simulink model "LQR_sim_discrete"  (R2020b)
settings: Solver=FixedStepAuto  StartTime=0.0  StopTime=60  FixedStep=0.0001  RelTol=1e-3  EnableMultiTasking=on
values from neighbouring files (symbols this model uses):
  Theta1_0 = pi    (= 3.14159265359)    [simulation.m]
  Theta2_0 = -pi/2    (= -1.57079632679)    [simulation.m]
  Thetad1_0 = 0    [simulation.m]
  Thetad2_0 = 0    [simulation.m]
undefined symbols (not defined in the file or in its folder): Discrete, h, Kd, Q, R, Time
libraries: simulink x4, ctrlSharedLib x1
settings Model: Creator=rbabuska  LastModifiedBy=fabia
settings SolverCC: AutoInsertRateTranBlk=on
settings DataIOCC: LimitDataPoints=on  SaveFormat=Array  ReturnWorkspaceOutputs=off  SignalLoggingName=sigsOut
settings OptimizationCC: BooleanDataType=off  ExpressionDepthLimit=2147483647  InitFltsAndDblsToZero=on  LifeSpan=inf
settings DebuggingCC: SaveWithParameterizedLinksMsg=none  SignalResolutionControl=TryResolveAllWithWarning  MultiTaskDSMMsg=warning  MultiTaskCondExecSysMsg=none  AllowSymbolicDim=off  StateNameClashWarn=warning  SFUnexpectedBacktrackingDiag=warning  SFNoUnconditionalDefaultTransitionDiag=warning  SFExecutionAtInitializationDiag=none  ArithmeticOperatorsInVariantConditions=warning
settings HardwareCC: ProdBitPerPointer=32  ProdBitPerSizeT=32  ProdBitPerPtrDiffT=32  ProdLargestAtomicFloat=None  ProdIntDivRoundTo=Undefined  ProdEndianess=Unspecified  ProdWordSize=32  ProdHWDeviceType=32-bit Generic  TargetUnknown=on
settings ModelReferenceCC: PropagateSignalLabelsOutOfModel=off
settings SFSimCC: SimUseLocalCustomCode=off  CustomCodeUndefinedFunction=UseInterfaceOnly
settings RTWCC: RTWUseLocalCustomCode=off
settings CodeAppCC: StateflowObjectComments=on
settings GRTTargetCC: TargetFcnLib=ansi_tfl_tmw.mat  TargetLangStandard=C89/C90 (ANSI)  CombineOutputUpdateFcns=off  GRTInterface=on
settings ConfigComp: CovMetricSettings=dw  CovSaveCumulativeToWorkspaceVar=on  CovSaveSingleToWorkspaceVar=on  CovExternalEMLEnable=off

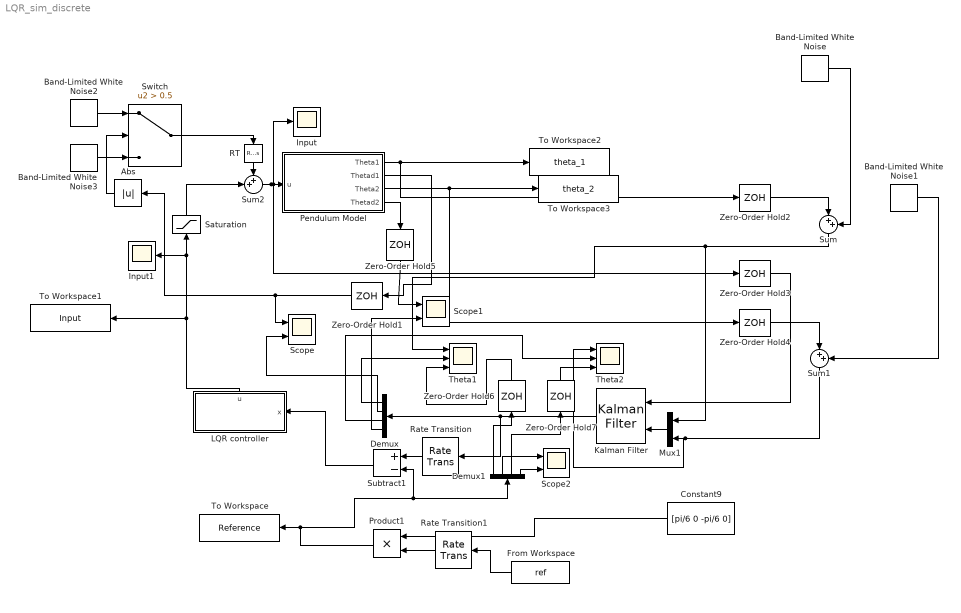
== system LQR_sim_discrete ==
  Abs : Abs
  Band-Limited White Noise : simulink/Sources/Band-Limited White Noise  Cov=R(1,1) * h  Ts=h  seed=[23341]
  Band-Limited White Noise1 : simulink/Sources/Band-Limited White Noise  Cov=R(2,2) * h  Ts=h  seed=[23546]
  Band-Limited White Noise2 : simulink/Sources/Band-Limited White Noise  Cov=Q*h  Ts=0.01  seed=[23341]
  Band-Limited White Noise3 : simulink/Sources/Band-Limited White Noise  Cov=Q*5  Ts=0.01  seed=[23341]
  Constant9 : Constant  Value=[pi/6 0 -pi/6 0]
  Demux : Demux
  Demux1 : Demux
  From Workspace : FromWorkspace  VariableName=ref  SampleTime=h
  Input : Scope
  Input1 : Scope
  Kalman Filter : ctrlSharedLib/Kalman Filter  TimeDomain=Discrete-Time  UseCurrentEstimator=on  ModelSource=LTI State-Space Variable  ModelSourceVariable=sysd  A=0.95  B=1  C=1  D=0  NumberOfStates=1  NumberOfInputs=1  NumberOfOutputs=1  InitialEstimateSource=Dialog  X0=0  P0=10  UseK=off  UseGH=off  NumberOfProcessNoiseInputs=1  G=1  TimeInvariantG=on  H=0  TimeInvariantH=on  Q=Q  TimeInvariantQ=on  R=R  TimeInvariantR=on  N=0  TimeInvariantN=on  AddInputPort=on  AddEnablePort=off  OutputEstimatedY=off  OutputP=off  Ts=-1
  LQR controller : Subsystem
      settings: PortSchema="{\"entries\":[{\"content\":{\"sides\":[{\"content\":{\"connectorIds\":[\"In1\"]},\"type\":\"ConnectorPlacement.EquallySpacedRectSide\",\"uuid\":\"a829bb76-8c32-4efb-bc1d-6bbdd337957d\"},{\"content\":{\"connectorIds\":[],\"side\":\"RIGHT\"},\"type\":\"ConnectorPlacement.EquallySpacedRectSide\",\"uuid\":\"eecab09d-eb4e-4271-bbad-67f1ecd3f7cb\"},{\"content\":{\"connectorIds\":[\"Out1\"],\"side\":\"TOP\"},\"type\":\"ConnectorPlacement.EquallySpacedRectSide\",\"uuid\":\"cb69e62e-93af-466c-bc77-09ee124a36c9\"},{\"content\":{\"connectorIds\":[],\"side\":\"HIDDEN\"},\"type\":\"ConnectorPlacement.EquallySpacedRectSide\",\"uuid\":\"8cf3d3f7-c3b5-449a-9c77-3afa19a1a637\"}]},\"type\":\"ConnectorPlacement.EquallySpacedConnector\",\"uuid\":\"e69d0e99-04d0-49a4-bcc0-927adbe84b1d\"}],\"packageUris\":[\"http://schema.mathworks.com/mf0/Connector/R2020b\"],\"version\":\"1.0\"}"
  Mux1 : Mux  Inputs=2
  Pendulum Model : Subsystem
  Product1 : Product
  RT : RateTransition  OutPortSampleTime=0.0001
  Rate Transition : RateTransition
  Rate Transition1 : RateTransition
  Saturation : Saturate  UpperLimit=1  LowerLimit=-1
  Scope : Scope  NumInputPorts=2
  Scope1 : Scope  NumInputPorts=2
  Scope2 : Scope  NumInputPorts=2
  Subtract1 : Sum  Inputs=+-
  Sum : Sum  Inputs=|++
  Sum1 : Sum  Inputs=|++
  Sum2 : Sum  Inputs=++|
  Switch : Switch  Criteria=u2 > Threshold  Threshold=0.5
  Theta1 : Scope  NumInputPorts=3
  Theta2 : Scope  NumInputPorts=3
  To Workspace : ToWorkspace  VariableName=Reference  SaveFormat=Timeseries  SampleTime=-1
  To Workspace1 : ToWorkspace  VariableName=Input  SaveFormat=Timeseries  SampleTime=-1
  To Workspace2 : ToWorkspace  VariableName=theta_1  SaveFormat=Timeseries  SampleTime=-1
  To Workspace3 : ToWorkspace  VariableName=theta_2  SaveFormat=Timeseries  SampleTime=-1
  Zero-Order Hold{1..7} (7 alike) : ZeroOrderHold  SampleTime=h
  wires:
  Pendulum Model/1(Theta1) -> To Workspace2/1, Zero-Order Hold2/1
  Pendulum Model/3(Theta2) -> Zero-Order Hold4/1, To Workspace3/1
  Zero-Order Hold3/1 -> Kalman Filter/1
  Band-Limited White Noise/1 -> Sum/2
  Zero-Order Hold2/1 -> Sum/1
  Sum/1 -> Theta1/1, Mux1/1
  Mux1/1 -> Kalman Filter/2
  Zero-Order Hold4/1 -> Sum1/1
  Sum1/1 -> Theta2/1, Mux1/2
  Band-Limited White Noise1/1 -> Sum1/2
  Saturation/1 -> Sum2/2
  Sum2/1 -> Input/1, Zero-Order Hold3/1, Pendulum Model/1(u)
  From Workspace/1 -> Rate Transition1/1
  Constant9/1 -> Product1/1
  Kalman Filter/1 -> Rate Transition/1, Demux/1
  Subtract1/1 -> LQR controller/1(x)
  Demux/1 -> Theta1/2
  Demux1/1 -> Zero-Order Hold6/1
  Demux/3 -> Theta2/2
  Demux1/3 -> Zero-Order Hold7/1
  Demux/4 -> Scope1/2
  Pendulum Model/4(Thetad2) -> Zero-Order Hold5/1
  Pendulum Model/2(Thetad1) -> Zero-Order Hold1/1
  LQR controller/1(u) -> Saturation/1, Input1/1, To Workspace1/1
  Band-Limited White Noise3/1 -> Switch/3
  Band-Limited White Noise2/1 -> Switch/1
  Abs/1 -> Switch/2
  Switch/1 -> RT/1
  Zero-Order Hold1/1 -> Scope/1, Abs/1
  Demux1/2 -> Scope2/1
  Demux1/4 -> Scope2/2
  Demux/2 -> Scope/2
  Zero-Order Hold5/1 -> Scope1/1
  Zero-Order Hold6/1 -> Theta1/3
  Zero-Order Hold7/1 -> Theta2/3
  Rate Transition/1 -> Subtract1/1
  RT/1 -> Sum2/1
  Product1/1 -> Demux1/1, Subtract1/2, To Workspace/1
  Rate Transition1/1 -> Product1/2

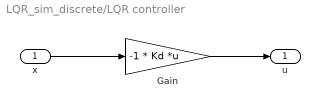
== system LQR_sim_discrete/LQR controller ==
  x : Inport
  Gain : Gain  Gain=-1 * Kd  Multiplication=Matrix(K*u) (u vector)
  u : Outport
  wires:
  x/1 -> Gain/1
  Gain/1 -> u/1

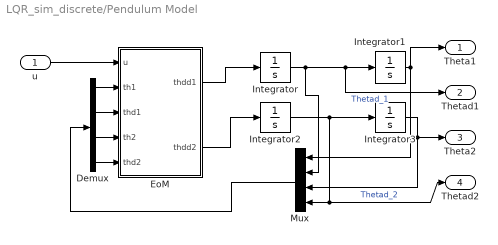
== system LQR_sim_discrete/Pendulum Model ==
  u : Inport
  Demux : Demux
  EoM : MATLAB Function  TreatAsAtomicUnit=on
  Integrator : Integrator  InitialCondition=Thetad1_0  ContinuousStateAttributes='Theta1'
  Integrator1 : Integrator  InitialCondition=Theta1_0  ContinuousStateAttributes='Theta1'
  Integrator2 : Integrator  InitialCondition=Thetad2_0  ContinuousStateAttributes='Theta1'
  Integrator3 : Integrator  InitialCondition=Theta2_0  ContinuousStateAttributes='Theta1'
  Mux : Mux
  Theta1 : Outport
  Thetad1 : Outport  Port=2
  Theta2 : Outport  Port=3
  Thetad2 : Outport  Port=4
  wires:
  Integrator1/1 -> Mux/1, Theta1/1
  Integrator/1 -> Mux/2, Integrator1/1, Thetad1/1  "Thetad_1"
  EoM/2(thdd2) -> Integrator2/1
  Integrator2/1 -> Thetad2/1, Mux/4, Integrator3/1  "Thetad_2"
  Integrator3/1 -> Theta2/1, Mux/3
  u/1 -> EoM/1(u)
  EoM/1(thdd1) -> Integrator/1
  Demux/1 -> EoM/2(th1)
  Demux/2 -> EoM/3(thd1)
  Demux/3 -> EoM/4(th2)
  Demux/4 -> EoM/5(thd2)
  Mux/1 -> Demux/1

== matlab function LQR_sim_discrete/Pendulum Model/EoM ==
  data: u input; thdd1 output; th1 input; thd1 input; th2 input; thd2 input; model_par parameter; thdd2 output
function [thdd1, thdd2] = fcn(u, th1, thd1, th2, thd2, model_par)
thdd1 = -model_par.a11*thd1 - model_par.a12 * u;
F = -model_par.c2*model_par.l1*model_par.m2*sin(thd2)*thd1^2 - model_par.b2*thd2 + model_par.c2*model_par.g*model_par.m2*sin(th1 + th2);
M21 = model_par.m2*model_par.c2^2 + model_par.l1*model_par.m2*cos(thd2)*model_par.c2 + model_par.J2;
M22 = model_par.m2*model_par.c2^2 + model_par.J2;
thdd2 = F/M22 - M21/M22 * thdd1;
